simulink model "cable_trim"  (R2024b)
settings: configuration reference "prj_default_config" (kept outside this file)
undefined symbols (not defined in the file): CONTROL_CONST, CONTROL_PARAM
libraries: mqlib x3
settings Model: Creator=yangyu  LastModifiedBy=yangyu
settings ConfigSetRef: SourceName=prj_default_config  SourceLocation=Base Workspace

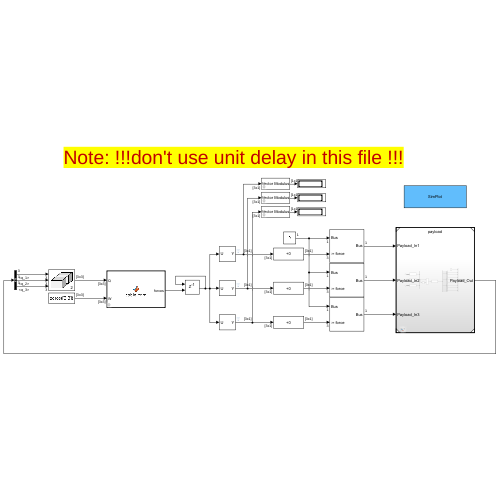
[thumbnail: Simulink's stored preview of the top-level diagram]
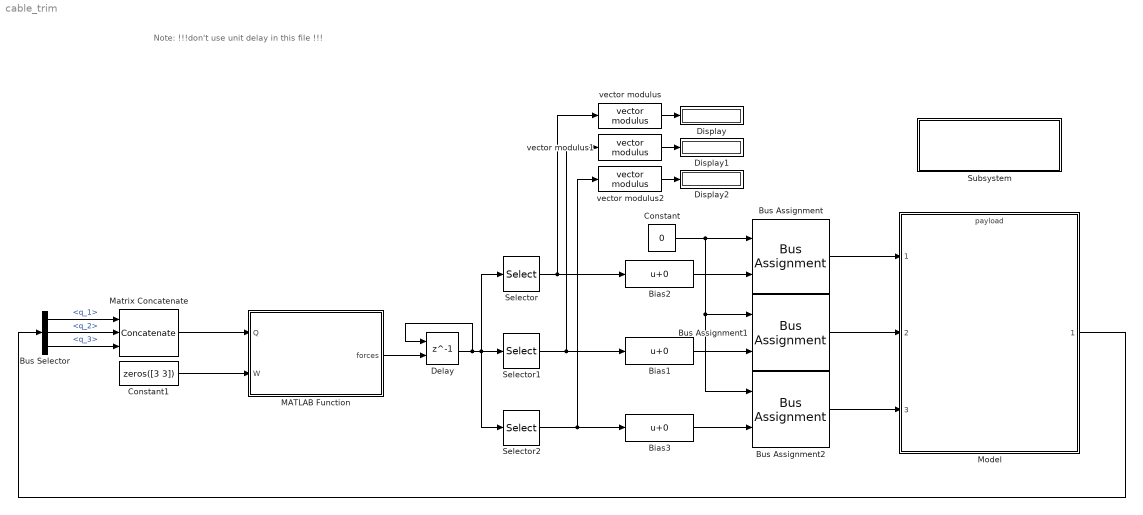
== system cable_trim ==
  note: Note: !!!don't use unit delay in this file !!!
  Bias1 : Bias  SaturateOnIntegerOverflow=off
  Bias2 : Bias  SaturateOnIntegerOverflow=off
  Bias3 : Bias  SaturateOnIntegerOverflow=off
  Bus Assignment : BusAssignment  AssignedSignals=force
  Bus Assignment1 : BusAssignment  AssignedSignals=force
  Bus Assignment2 : BusAssignment  AssignedSignals=force
  Bus Selector : BusSelector  OutputSignals=q_1,q_2,q_3
  Constant : Constant  Value=0  OutDataTypeStr=Bus: Payload_In_Bus
  Constant1 : Constant  Value=zeros([3 3])
  Delay : Delay  DelayLength=1  InitialConditionSource=Input port
      settings: InputPortMap=u0,p4
  Display : Display
  Display1 : Display
  Display2 : Display
  MATLAB Function : MATLAB Function  TreatAsAtomicUnit=on  mask{mL=CONTROL_PARAM.MASS_LOAD, M=CONTROL_PARAM.MASS_UAV * ones(3,1), L=CONTROL_PARAM.CABLE_LEN * ones(3,1), g=CONTROL_CONST.g}
  Matrix Concatenate : Concatenate  NumInputs=3  Mode=Multidimensional array  ConcatenateDimension=2
  Model : ModelReference  ModelNameDialog=payload.slx  SimulationMode=Normal  ModelReferenceVersion=1.90
  Selector : Selector  NumberOfDimensions=2  InputPortWidth=3  IndexOptions=Index vector (dialog),Index vector (dialog)  Indices=[1 2 3],[1]  OutputSizes=1,1
  Selector1 : Selector  NumberOfDimensions=2  InputPortWidth=3  IndexOptions=Index vector (dialog),Index vector (dialog)  Indices=[1 2 3],[2]  OutputSizes=1,1
  Selector2 : Selector  NumberOfDimensions=2  InputPortWidth=3  IndexOptions=Index vector (dialog),Index vector (dialog)  Indices=[1 2 3],[3]  OutputSizes=1,1
  Subsystem : Subsystem
      settings: OpenFcn=run('simplot.m');
      mask Display: disp('SimPlot');
  vector modulus : mqlib/vector modulus
  vector modulus1 : mqlib/vector modulus
  vector modulus2 : mqlib/vector modulus
  wires:
  Constant/1 -> Bus Assignment1/1, Bus Assignment2/1, Bus Assignment/1
  Bus Assignment/1 -> Model/1
  Model/1 -> Bus Selector/1
  Delay/1 -> Delay/1, Selector1/1, Selector/1, Selector2/1
  Constant1/1 -> MATLAB Function/2(W)
  Bus Selector/1 -> Matrix Concatenate/1  "<q_1>"
  Bus Selector/2 -> Matrix Concatenate/2  "<q_2>"
  Bus Selector/3 -> Matrix Concatenate/3  "<q_3>"
  Matrix Concatenate/1 -> MATLAB Function/1(Q)
  Bus Assignment1/1 -> Model/2
  Bus Assignment2/1 -> Model/3
  MATLAB Function/1(forces) -> Delay/2
  Selector/1 -> Bias2/1, vector modulus/1
  Selector2/1 -> Bias3/1, vector modulus2/1
  Bias1/1 -> Bus Assignment1/2
  Bias3/1 -> Bus Assignment2/2
  Bias2/1 -> Bus Assignment/2
  vector modulus/1 -> Display/1
  vector modulus1/1 -> Display1/1
  vector modulus2/1 -> Display2/1
  Selector1/1 -> Bias1/1, vector modulus1/1

== system cable_trim/Subsystem ==

== matlab function cable_trim/MATLAB Function ==
  data: forces output; Q input; W input; mL parameter; M parameter; L parameter; g parameter
function forces  = cable_trim(Q, W, mL, M, L, g)
% mL: mass of payload (scalar)
% M: drone mass vector (3 X 1)
% L: length vector of cables (3 X 1)
% Q: cable direction matrix (3 X 3)
% W: cable angular velocity matrix (3 X 3)
g = [0; 0; 9.8];
Fd = mL * -g;
vu = Q' / (Q * Q') * Fd;
ui_parallel = zeros([3 3]);
ui_vertical = zeros([3 3]);

for i = 1:3
    mi = M(i);
    li = L(i);
    qi = Q(:, i);
    wi = W(:, i);
    ai = -g;
    ui_parallel(:, i) = vu(i) * qi + mi * li * norm(wi) ^ 2 * qi + mi * qi * qi' * ai;
    Sqi = [0 -qi(3) qi(2); qi(3) 0 -qi(1); -qi(2) qi(1) 0];
    % null space
    % ui_vertical(:, i) = mi * (ai + k * qi), qi is the base of null space.
    % let k*qi = -q*q'*a.
    ui_vertical(:, i) = -mi * Sqi * Sqi * ai;
end

forces = ui_parallel + ui_vertical;
end
